simulink model "rep3_transc_analysis_fullmodel_combo"  (R2015a)
settings: Solver=ode4  StartTime=0.0  StopTime=1500  FixedStep=0.1  RelTol=1e-3
values from neighbouring files (symbols this model uses):
  c1 = 1.6    [rep3_transc_analysis_init.m]
  c2 = 0.12    [rep3_transc_analysis_init.m]
  c3 = 2.6    [rep3_transc_analysis_init.m]
  c4 = 0.06    [rep3_transc_analysis_init.m]
  mRNA_init = 0.5    [rep3_transc_analysis_init.m]
libraries: fuzblock x6
settings Model: Creator=Jure Bordon  LastModifiedBy=jure
settings DataIOCC: InspectSignalLogs=on
settings DebuggingCC: UnderspecifiedInitializationDetection=Classic  MergeDetectMultiDrivingBlocksExec=none  SolverPrmCheckMsg=warning  StateNameClashWarn=warning

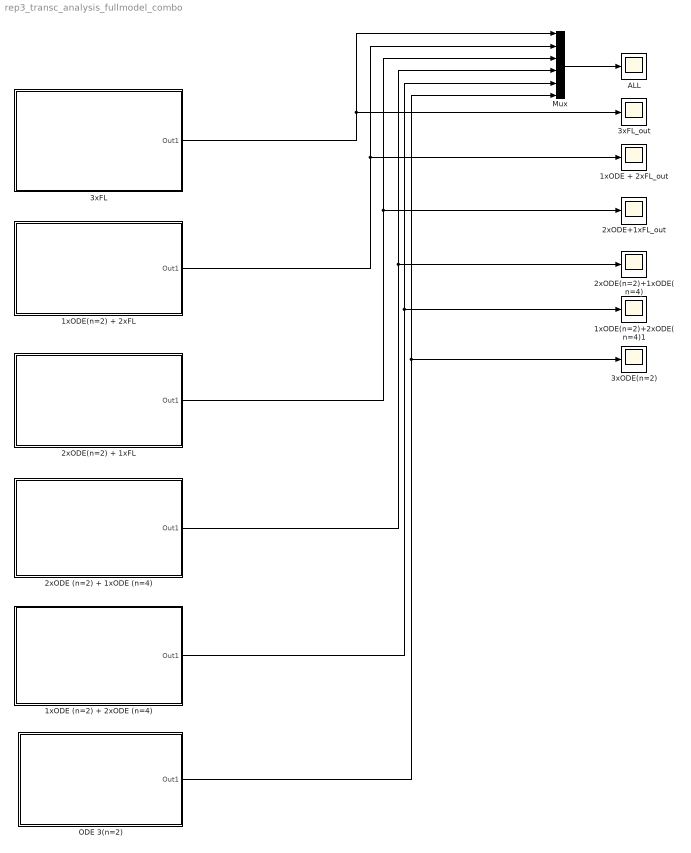
== system rep3_transc_analysis_fullmodel_combo ==
  1xODE (n=2) + 2xODE (n=4) : Subsystem
  1xODE + 2xFL_out : Scope
      settings: TimeRange=1500  YMin=0  YMax=450  SaveName=P_out_FL5
  1xODE(n=2) + 2xFL : Subsystem
  1xODE(n=2)+2xODE(n=4)1 : Scope
      settings: TimeRange=1500  YMin=0  YMax=600  SaveName=P_out_FL6
  2xODE (n=2) + 1xODE (n=4) : Subsystem
  2xODE(n=2) + 1xFL : Subsystem
  2xODE(n=2)+1xODE(n=4) : Scope
      settings: TimeRange=1500  YMin=0  YMax=600  SaveName=P_out_FL2
  2xODE+1xFL_out : Scope
      settings: TimeRange=1500  YMin=0  YMax=500  SaveName=P_out_FL1
  3xFL : Subsystem
  3xFL_out : Scope
      settings: TimeRange=1500  YMin=0  YMax=450  SaveName=P_out_FL
  3xODE(n=2) : Scope
      settings: TimeRange=1500  YMin=0  YMax=400  SaveName=P_out_FL3
  ALL : Scope
      settings: TimeRange=1500  YMin=0  YMax=500  SaveName=P_out_FL4
  Mux : Mux  Inputs=6
  ODE 3(n=2) : Subsystem
  wires:
  2xODE (n=2) + 1xODE (n=4)/1(Out1) -> Mux/4, 2xODE(n=2)+1xODE(n=4)/1
  2xODE(n=2) + 1xFL/1(Out1) -> Mux/3, 2xODE+1xFL_out/1
  ODE 3(n=2)/1(Out1) -> Mux/6, 3xODE(n=2)/1
  Mux/1 -> ALL/1
  3xFL/1(Out1) -> 3xFL_out/1, Mux/1
  1xODE(n=2) + 2xFL/1(Out1) -> 1xODE + 2xFL_out/1, Mux/2
  1xODE (n=2) + 2xODE (n=4)/1(Out1) -> Mux/5, 1xODE(n=2)+2xODE(n=4)1/1

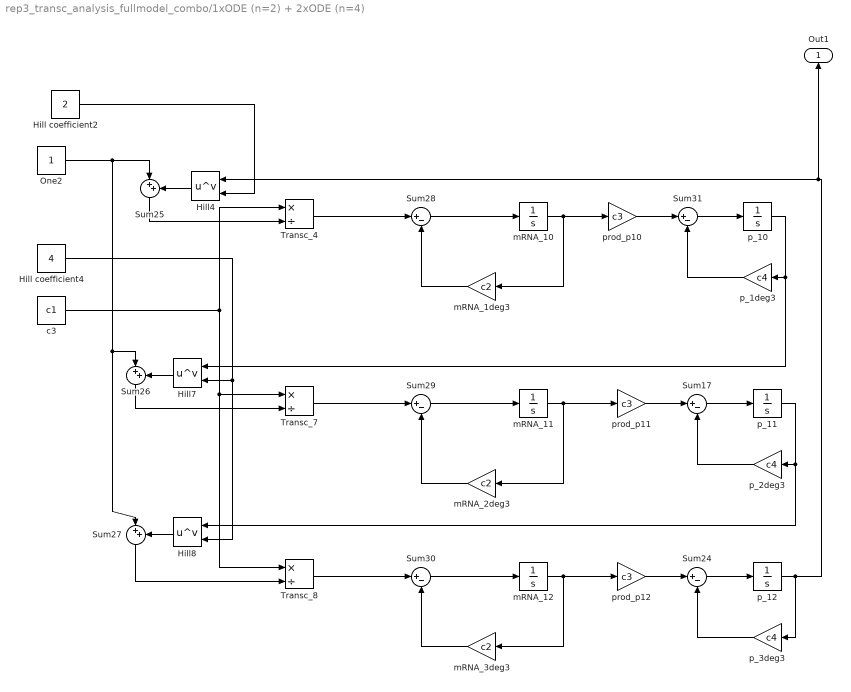
== system rep3_transc_analysis_fullmodel_combo/1xODE (n=2) + 2xODE (n=4) ==
  Hill coefficient2 : Constant  Value=2
  Hill coefficient4 : Constant  Value=4
  Hill4 : Math  Operator=pow  SaturateOnIntegerOverflow=on
  Hill7 : Math  Operator=pow  SaturateOnIntegerOverflow=on
  Hill8 : Math  Operator=pow  SaturateOnIntegerOverflow=on
  One2 : Constant
  Sum{17,24,28..31} (6 alike) : Sum  Inputs=|+-
  Sum25 : Sum  Inputs=|++
  Sum26 : Sum  Inputs=|++
  Sum27 : Sum  Inputs=|++
  Transc_4 : Product  Inputs=*/
  Transc_7 : Product  Inputs=*/
  Transc_8 : Product  Inputs=*/
  c3 : Constant  Value=c1
  mRNA_10 : Integrator  InitialCondition=mRNA_init + 0.5
  mRNA_11 : Integrator  InitialCondition=mRNA_init
  mRNA_12 : Integrator  InitialCondition=mRNA_init
  mRNA_1deg3 : Gain  Gain=c2
  mRNA_2deg3 : Gain  Gain=c2
  mRNA_3deg3 : Gain  Gain=c2
  p_10 : Integrator
  p_11 : Integrator
  p_12 : Integrator
  p_1deg3 : Gain  Gain=c4
  p_2deg3 : Gain  Gain=c4
  p_3deg3 : Gain  Gain=c4
  prod_p10 : Gain  Gain=c3
  prod_p11 : Gain  Gain=c3
  prod_p12 : Gain  Gain=c3
  Out1 : Outport
  wires:
  Sum31/1 -> p_10/1
  p_1deg3/1 -> Sum31/2
  Sum17/1 -> p_11/1
  p_11/1 -> p_2deg3/1, Hill8/1
  p_10/1 -> Hill7/1, p_1deg3/1
  Sum29/1 -> mRNA_11/1
  Sum28/1 -> mRNA_10/1
  Sum30/1 -> mRNA_12/1
  Sum24/1 -> p_12/1
  p_3deg3/1 -> Sum24/2
  mRNA_10/1 -> prod_p10/1, mRNA_1deg3/1
  mRNA_11/1 -> prod_p11/1, mRNA_2deg3/1
  Transc_7/1 -> Sum29/1
  Sum25/1 -> Transc_4/2
  p_2deg3/1 -> Sum17/2
  mRNA_12/1 -> mRNA_3deg3/1, prod_p12/1
  p_12/1 -> p_3deg3/1, Out1/1, Hill4/1
  One2/1 -> Sum26/1, Sum27/1, Sum25/1
  Transc_8/1 -> Sum30/1
  Sum26/1 -> Transc_7/2
  Sum27/1 -> Transc_8/2
  c3/1 -> Transc_4/1, Transc_8/1, Transc_7/1
  prod_p12/1 -> Sum24/1
  mRNA_1deg3/1 -> Sum28/2
  prod_p11/1 -> Sum17/1
  prod_p10/1 -> Sum31/1
  Hill7/1 -> Sum26/2
  Transc_4/1 -> Sum28/1
  Hill4/1 -> Sum25/2
  Hill8/1 -> Sum27/2
  mRNA_2deg3/1 -> Sum29/2
  Hill coefficient4/1 -> Hill8/2, Hill7/2
  Hill coefficient2/1 -> Hill4/2
  mRNA_3deg3/1 -> Sum30/2

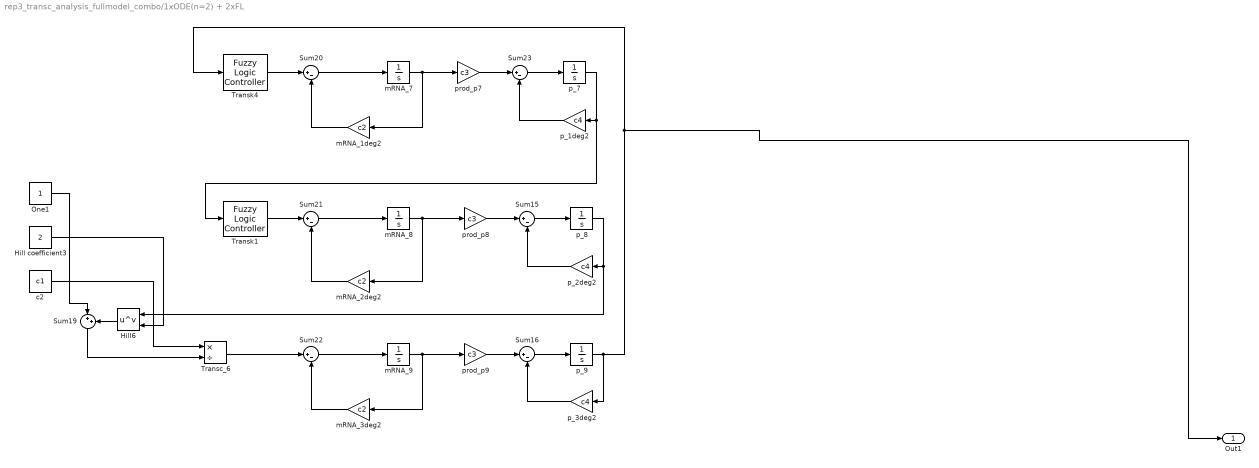
== system rep3_transc_analysis_fullmodel_combo/1xODE(n=2) + 2xFL ==
  Hill coefficient3 : Constant  Value=2
  Hill6 : Math  Operator=pow  SaturateOnIntegerOverflow=on
  One1 : Constant
  Sum{15..16,20..23} (6 alike) : Sum  Inputs=|+-
  Sum19 : Sum  Inputs=|++
  Transc_6 : Product  Inputs=*/
  Transk1 : fuzblock/Fuzzy Logic  Controller  fis=Transk1
  Transk4 : fuzblock/Fuzzy Logic  Controller  fis=Transk1
  c2 : Constant  Value=c1
  mRNA_1deg2 : Gain  Gain=c2
  mRNA_2deg2 : Gain  Gain=c2
  mRNA_3deg2 : Gain  Gain=c2
  mRNA_7 : Integrator  InitialCondition=mRNA_init + 0.5
  mRNA_8 : Integrator  InitialCondition=mRNA_init
  mRNA_9 : Integrator  InitialCondition=mRNA_init
  p_1deg2 : Gain  Gain=c4
  p_2deg2 : Gain  Gain=c4
  p_3deg2 : Gain  Gain=c4
  p_7 : Integrator
  p_8 : Integrator
  p_9 : Integrator
  prod_p7 : Gain  Gain=c3
  prod_p8 : Gain  Gain=c3
  prod_p9 : Gain  Gain=c3
  Out1 : Outport
  wires:
  p_3deg2/1 -> Sum16/2
  prod_p7/1 -> Sum23/1
  Sum23/1 -> p_7/1
  p_1deg2/1 -> Sum23/2
  p_9/1 -> p_3deg2/1, Out1/1, Transk4/1
  mRNA_9/1 -> mRNA_3deg2/1, prod_p9/1
  mRNA_3deg2/1 -> Sum22/2
  p_2deg2/1 -> Sum15/2
  mRNA_2deg2/1 -> Sum21/2
  mRNA_7/1 -> prod_p7/1, mRNA_1deg2/1
  Sum16/1 -> p_9/1
  Transk1/1 -> Sum21/1
  prod_p8/1 -> Sum15/1
  p_7/1 -> Transk1/1, p_1deg2/1
  One1/1 -> Sum19/1
  Sum19/1 -> Transc_6/2
  mRNA_8/1 -> prod_p8/1, mRNA_2deg2/1
  Transc_6/1 -> Sum22/1
  Sum20/1 -> mRNA_7/1
  prod_p9/1 -> Sum16/1
  p_8/1 -> p_2deg2/1, Hill6/1
  Sum22/1 -> mRNA_9/1
  Sum15/1 -> p_8/1
  Sum21/1 -> mRNA_8/1
  c2/1 -> Transc_6/1
  mRNA_1deg2/1 -> Sum20/2
  Hill6/1 -> Sum19/2
  Hill coefficient3/1 -> Hill6/2
  Transk4/1 -> Sum20/1

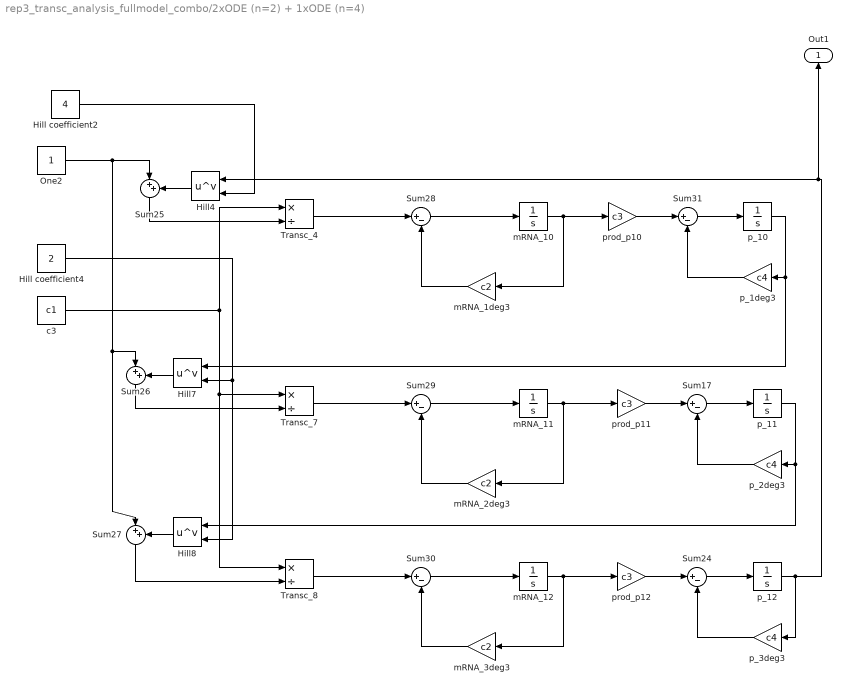
== system rep3_transc_analysis_fullmodel_combo/2xODE (n=2) + 1xODE (n=4) ==
  Hill coefficient2 : Constant  Value=4
  Hill coefficient4 : Constant  Value=2
  Hill4 : Math  Operator=pow  SaturateOnIntegerOverflow=on
  Hill7 : Math  Operator=pow  SaturateOnIntegerOverflow=on
  Hill8 : Math  Operator=pow  SaturateOnIntegerOverflow=on
  One2 : Constant
  Sum{17,24,28..31} (6 alike) : Sum  Inputs=|+-
  Sum25 : Sum  Inputs=|++
  Sum26 : Sum  Inputs=|++
  Sum27 : Sum  Inputs=|++
  Transc_4 : Product  Inputs=*/
  Transc_7 : Product  Inputs=*/
  Transc_8 : Product  Inputs=*/
  c3 : Constant  Value=c1
  mRNA_10 : Integrator  InitialCondition=mRNA_init + 0.5
  mRNA_11 : Integrator  InitialCondition=mRNA_init
  mRNA_12 : Integrator  InitialCondition=mRNA_init
  mRNA_1deg3 : Gain  Gain=c2
  mRNA_2deg3 : Gain  Gain=c2
  mRNA_3deg3 : Gain  Gain=c2
  p_10 : Integrator
  p_11 : Integrator
  p_12 : Integrator
  p_1deg3 : Gain  Gain=c4
  p_2deg3 : Gain  Gain=c4
  p_3deg3 : Gain  Gain=c4
  prod_p10 : Gain  Gain=c3
  prod_p11 : Gain  Gain=c3
  prod_p12 : Gain  Gain=c3
  Out1 : Outport
  wires:
  Sum31/1 -> p_10/1
  p_1deg3/1 -> Sum31/2
  Sum17/1 -> p_11/1
  p_11/1 -> p_2deg3/1, Hill8/1
  p_10/1 -> Hill7/1, p_1deg3/1
  Sum29/1 -> mRNA_11/1
  Sum28/1 -> mRNA_10/1
  Sum30/1 -> mRNA_12/1
  Sum24/1 -> p_12/1
  p_3deg3/1 -> Sum24/2
  mRNA_10/1 -> prod_p10/1, mRNA_1deg3/1
  mRNA_11/1 -> prod_p11/1, mRNA_2deg3/1
  Transc_7/1 -> Sum29/1
  Sum25/1 -> Transc_4/2
  p_2deg3/1 -> Sum17/2
  mRNA_12/1 -> mRNA_3deg3/1, prod_p12/1
  p_12/1 -> p_3deg3/1, Out1/1, Hill4/1
  One2/1 -> Sum26/1, Sum27/1, Sum25/1
  Transc_8/1 -> Sum30/1
  Sum26/1 -> Transc_7/2
  Sum27/1 -> Transc_8/2
  c3/1 -> Transc_4/1, Transc_8/1, Transc_7/1
  prod_p12/1 -> Sum24/1
  mRNA_1deg3/1 -> Sum28/2
  prod_p11/1 -> Sum17/1
  prod_p10/1 -> Sum31/1
  Hill7/1 -> Sum26/2
  Transc_4/1 -> Sum28/1
  Hill4/1 -> Sum25/2
  Hill8/1 -> Sum27/2
  mRNA_2deg3/1 -> Sum29/2
  Hill coefficient4/1 -> Hill8/2, Hill7/2
  Hill coefficient2/1 -> Hill4/2
  mRNA_3deg3/1 -> Sum30/2

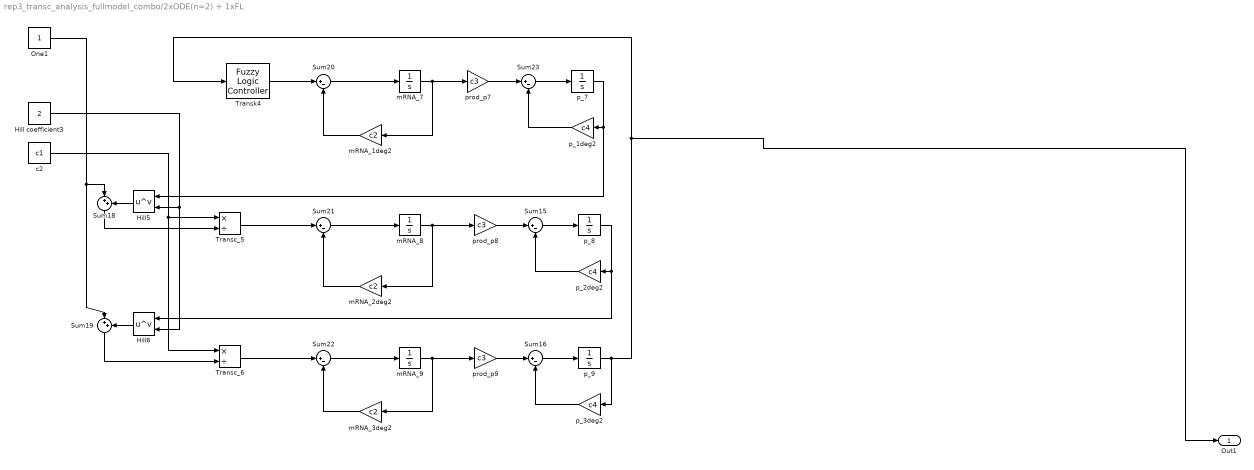
== system rep3_transc_analysis_fullmodel_combo/2xODE(n=2) + 1xFL ==
  Hill coefficient3 : Constant  Value=2
  Hill5 : Math  Operator=pow  SaturateOnIntegerOverflow=on
  Hill6 : Math  Operator=pow  SaturateOnIntegerOverflow=on
  One1 : Constant
  Sum{15..16,20..23} (6 alike) : Sum  Inputs=|+-
  Sum18 : Sum  Inputs=|++
  Sum19 : Sum  Inputs=|++
  Transc_5 : Product  Inputs=*/
  Transc_6 : Product  Inputs=*/
  Transk4 : fuzblock/Fuzzy Logic  Controller  fis=Transk1
  c2 : Constant  Value=c1
  mRNA_1deg2 : Gain  Gain=c2
  mRNA_2deg2 : Gain  Gain=c2
  mRNA_3deg2 : Gain  Gain=c2
  mRNA_7 : Integrator  InitialCondition=mRNA_init + 0.5
  mRNA_8 : Integrator  InitialCondition=mRNA_init
  mRNA_9 : Integrator  InitialCondition=mRNA_init
  p_1deg2 : Gain  Gain=c4
  p_2deg2 : Gain  Gain=c4
  p_3deg2 : Gain  Gain=c4
  p_7 : Integrator
  p_8 : Integrator
  p_9 : Integrator
  prod_p7 : Gain  Gain=c3
  prod_p8 : Gain  Gain=c3
  prod_p9 : Gain  Gain=c3
  Out1 : Outport
  wires:
  p_3deg2/1 -> Sum16/2
  prod_p7/1 -> Sum23/1
  Hill5/1 -> Sum18/2
  Sum23/1 -> p_7/1
  p_1deg2/1 -> Sum23/2
  p_9/1 -> p_3deg2/1, Out1/1, Transk4/1
  mRNA_9/1 -> mRNA_3deg2/1, prod_p9/1
  mRNA_3deg2/1 -> Sum22/2
  Sum18/1 -> Transc_5/2
  p_2deg2/1 -> Sum15/2
  mRNA_2deg2/1 -> Sum21/2
  mRNA_7/1 -> prod_p7/1, mRNA_1deg2/1
  Sum16/1 -> p_9/1
  Transc_5/1 -> Sum21/1
  prod_p8/1 -> Sum15/1
  p_7/1 -> Hill5/1, p_1deg2/1
  One1/1 -> Sum18/1, Sum19/1
  Sum19/1 -> Transc_6/2
  mRNA_8/1 -> prod_p8/1, mRNA_2deg2/1
  Transc_6/1 -> Sum22/1
  Sum20/1 -> mRNA_7/1
  prod_p9/1 -> Sum16/1
  p_8/1 -> p_2deg2/1, Hill6/1
  Sum22/1 -> mRNA_9/1
  Sum15/1 -> p_8/1
  Sum21/1 -> mRNA_8/1
  c2/1 -> Transc_6/1, Transc_5/1
  mRNA_1deg2/1 -> Sum20/2
  Hill6/1 -> Sum19/2
  Hill coefficient3/1 -> Hill6/2, Hill5/2
  Transk4/1 -> Sum20/1

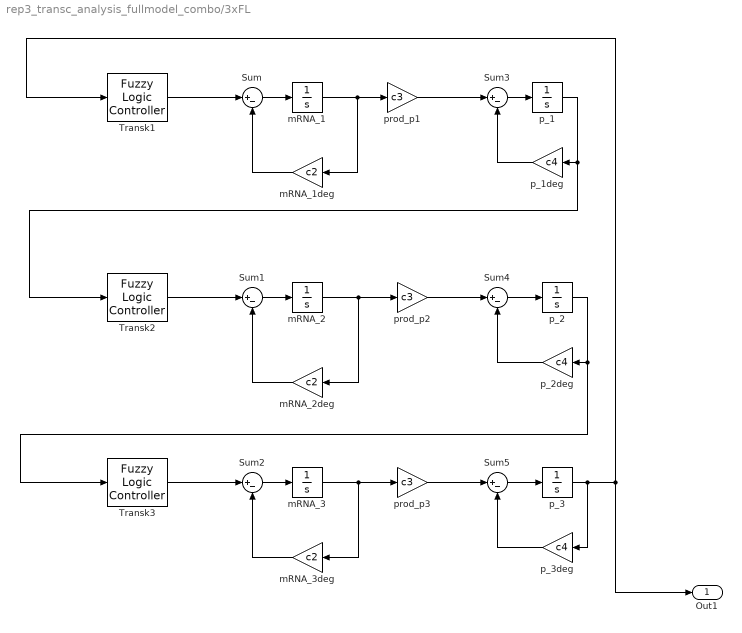
== system rep3_transc_analysis_fullmodel_combo/3xFL ==
  Sum{,1..5} (6 alike) : Sum  Inputs=|+-
  Transk1 : fuzblock/Fuzzy Logic  Controller  fis=Transk
  Transk2 : fuzblock/Fuzzy Logic  Controller  fis=Transk
  Transk3 : fuzblock/Fuzzy Logic  Controller  fis=Transk
  mRNA_1 : Integrator  InitialCondition=mRNA_init + 0.5  LimitOutput=on  LowerSaturationLimit=0
  mRNA_1deg : Gain  Gain=c2
  mRNA_2 : Integrator  InitialCondition=mRNA_init  LimitOutput=on  LowerSaturationLimit=0
  mRNA_2deg : Gain  Gain=c2
  mRNA_3 : Integrator  InitialCondition=mRNA_init  LimitOutput=on  LowerSaturationLimit=0
  mRNA_3deg : Gain  Gain=c2
  p_1 : Integrator  LimitOutput=on  LowerSaturationLimit=0
  p_1deg : Gain  Gain=c4
  p_2 : Integrator  LimitOutput=on  LowerSaturationLimit=0
  p_2deg : Gain  Gain=c4
  p_3 : Integrator  LimitOutput=on  LowerSaturationLimit=0
  p_3deg : Gain  Gain=c4
  prod_p1 : Gain  Gain=c3
  prod_p2 : Gain  Gain=c3
  prod_p3 : Gain  Gain=c3
  Out1 : Outport
  wires:
  Sum2/1 -> mRNA_3/1
  p_2deg/1 -> Sum4/2
  Sum5/1 -> p_3/1
  Sum4/1 -> p_2/1
  Sum1/1 -> mRNA_2/1
  Transk3/1 -> Sum2/1
  Transk2/1 -> Sum1/1
  Sum3/1 -> p_1/1
  p_1deg/1 -> Sum3/2
  p_3deg/1 -> Sum5/2
  Sum/1 -> mRNA_1/1
  mRNA_3/1 -> mRNA_3deg/1, prod_p3/1
  mRNA_1/1 -> prod_p1/1, mRNA_1deg/1
  mRNA_2/1 -> prod_p2/1, mRNA_2deg/1
  mRNA_2deg/1 -> Sum1/2
  mRNA_3deg/1 -> Sum2/2
  prod_p1/1 -> Sum3/1
  prod_p3/1 -> Sum5/1
  mRNA_1deg/1 -> Sum/2
  Transk1/1 -> Sum/1
  prod_p2/1 -> Sum4/1
  p_1/1 -> Transk2/1, p_1deg/1
  p_2/1 -> Transk3/1, p_2deg/1
  p_3/1 -> p_3deg/1, Out1/1, Transk1/1

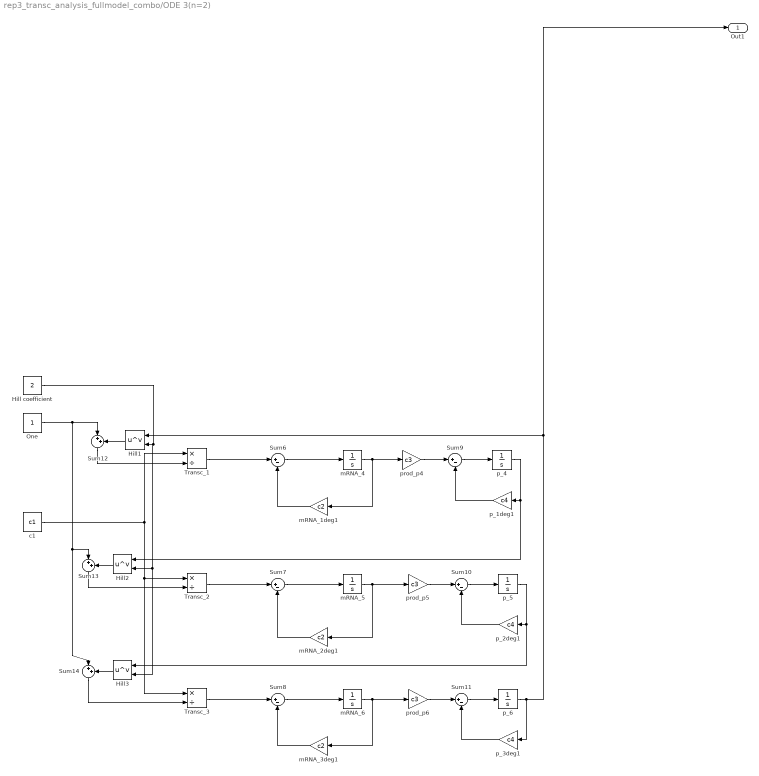
== system rep3_transc_analysis_fullmodel_combo/ODE 3(n=2) ==
  Hill coefficient : Constant  Value=2
  Hill1 : Math  Operator=pow  SaturateOnIntegerOverflow=on
  Hill2 : Math  Operator=pow  SaturateOnIntegerOverflow=on
  Hill3 : Math  Operator=pow  SaturateOnIntegerOverflow=on
  One : Constant
  Sum{6..11} (6 alike) : Sum  Inputs=|+-
  Sum12 : Sum  Inputs=|++
  Sum13 : Sum  Inputs=|++
  Sum14 : Sum  Inputs=|++
  Transc_1 : Product  Inputs=*/
  Transc_2 : Product  Inputs=*/
  Transc_3 : Product  Inputs=*/
  c1 : Constant  Value=c1
  mRNA_1deg1 : Gain  Gain=c2
  mRNA_2deg1 : Gain  Gain=c2
  mRNA_3deg1 : Gain  Gain=c2
  mRNA_4 : Integrator  InitialCondition=mRNA_init + 0.5
  mRNA_5 : Integrator  InitialCondition=mRNA_init
  mRNA_6 : Integrator  InitialCondition=mRNA_init
  p_1deg1 : Gain  Gain=c4
  p_2deg1 : Gain  Gain=c4
  p_3deg1 : Gain  Gain=c4
  p_4 : Integrator
  p_5 : Integrator
  p_6 : Integrator
  prod_p4 : Gain  Gain=c3
  prod_p5 : Gain  Gain=c3
  prod_p6 : Gain  Gain=c3
  Out1 : Outport
  wires:
  Transc_1/1 -> Sum6/1
  Hill coefficient/1 -> Hill3/2, Hill2/2, Hill1/2
  Sum10/1 -> p_5/1
  Sum11/1 -> p_6/1
  mRNA_3deg1/1 -> Sum8/2
  p_6/1 -> p_3deg1/1, Out1/1, Hill1/1
  mRNA_6/1 -> mRNA_3deg1/1, prod_p6/1
  Hill1/1 -> Sum12/2
  Transc_2/1 -> Sum7/1
  p_5/1 -> p_2deg1/1, Hill3/1
  mRNA_4/1 -> prod_p4/1, mRNA_1deg1/1
  p_2deg1/1 -> Sum10/2
  c1/1 -> Transc_1/1, Transc_3/1, Transc_2/1
  prod_p4/1 -> Sum9/1
  Sum6/1 -> mRNA_4/1
  mRNA_2deg1/1 -> Sum7/2
  prod_p6/1 -> Sum11/1
  Sum14/1 -> Transc_3/2
  p_3deg1/1 -> Sum11/2
  Sum12/1 -> Transc_1/2
  mRNA_5/1 -> prod_p5/1, mRNA_2deg1/1
  mRNA_1deg1/1 -> Sum6/2
  prod_p5/1 -> Sum10/1
  Sum9/1 -> p_4/1
  Hill2/1 -> Sum13/2
  p_4/1 -> Hill2/1, p_1deg1/1
  Sum13/1 -> Transc_2/2
  Sum8/1 -> mRNA_6/1
  Sum7/1 -> mRNA_5/1
  One/1 -> Sum13/1, Sum14/1, Sum12/1
  p_1deg1/1 -> Sum9/2
  Transc_3/1 -> Sum8/1
  Hill3/1 -> Sum14/2
